simulink model "sst"  (R2025a)
settings: Solver=ode1be  StartTime=0.0  StopTime=simlength  FixedStep=tc  MaxStep=ts_sim
values from neighbouring files (symbols this model uses):
  Adrso = eye(2) + Arso*ts_inv    [design_model.m]
  alpha = 35    [design_model.m]
  C1 = 0.5    [design_model.m]
  Crso = [1 0]    [design_model.m]
  DThs_init = 0    [design_model.m]
  E0 = 3.485    [design_model.m]
  E1 = 0.2156    [design_model.m]
  E2 = 0    [design_model.m]
  E3 = 0    [design_model.m]
  E_1 = -1.031    [design_model.m]
  Elog = -0.05    [design_model.m]
  fPWM_DAB = fPWM_INV    (= 35000)    [design_model.m]
  fPWM_INV = 35e3    (= 35000)    [design_model.m]
  freq = 50    [design_model.m]
  I_FS = Iout_ac_rms_nom * sqrt(2) * margin_factor    [design_model.m]
  ki_i_dab = 18    [design_model.m]
  ki_pll = 3140    [design_model.m]
  ki_v_dab = 45    [design_model.m]
  kp_i_dab = 2    [design_model.m]
  kp_pll = 314    [design_model.m]
  kp_v_dab = 8    [design_model.m]
  Ldrso = acker(Adrso',Crso',polesdrso)'    [design_model.m]
  M = 125    [design_model.m]
  number_of_cells = 30    [design_model.m]
  Q = 1000    [design_model.m]
  q1Kalman = ts_inv^2    (= 8.16326530612e-10)    [design_model.m]
  q2Kalman = ts_inv^1    (= 2.85714285714e-05)    [design_model.m]
  q3Kalman = 0    [design_model.m]
  R0 = 0.0035    [design_model.m]
  R1 = 0.0035    [design_model.m]
  rKalman = 1    [design_model.m]
  Tambient = 40    [design_model.m]
  tc = ts_inv/200    (= 1.42857142857e-07)    [design_model.m]
  ts_afe = ts_inv    (= 2.85714285714e-05)    [design_model.m]
  ts_dab = tPWM_DAB*2    (= 5.71428571429e-05)    [design_model.m]
  ts_inv = tPWM_INV    (= 2.85714285714e-05)    [design_model.m]
  V_FS = Vout_dc_nom * margin_factor    (= 500)    [design_model.m]
  weigth = 0.6/6    (= 0.1)    [design_model.m]
undefined symbols (not defined in the file or in its folder): Aresd, Bresd, Cresd, dead_time_DAB, dead_time_INV, iph_grid_pu_ref, ki_afe, kp_afe, LFu1_AFE, n_modules, omega_grid_nom, RLFu1_AFE, ts_battery, tsample, V_phase_normalization_factor, Vdab2_dc_nom
libraries: fl_lib x280, nesl_utility x188, ee_lib x41, cstblocks x4, single_phase_transformer_lib x2, lithium_ion_cell_lib x1, simulink x1
(part 1 of 12)
settings Model: SimulationMode=accelerator  Creator=LTNBDA  LastModifiedBy=dbagn
settings SolverCC: ZeroCrossControl=EnableAll  ZeroCrossAlgorithm=Adaptive  AlgebraicLoopSolver=TrustRegion  SolverResetMethod=Robust  AutoInsertRateTranBlk=on
settings DataIOCC: LimitDataPoints=on  MaxDataPoints=1  SaveFormat=Array  SignalLoggingSaveFormat=ModelDataLogs  SaveOutput=off  SignalLogging=off  DSMLogging=off  SaveTime=off  ReturnWorkspaceOutputs=off
settings OptimizationCC: ExpressionDepthLimit=2147483647.0  InitFltsAndDblsToZero=on  EfficientMapNaN2IntZero=off  LifeSpan=inf
settings DebuggingCC: SaveWithParameterizedLinksMsg=none  UnderspecifiedInitializationDetection=Classic  MergeDetectMultiDrivingBlocksExec=none  SignalResolutionControl=TryResolveAllWithWarning  SolverPrmCheckMsg=warning  MultiTaskDSMMsg=warning  MultiTaskCondExecSysMsg=none  MultiTaskRateTransMsg=warning  FcnCallInpInsideContextMsg=warning  StateNameClashWarn=warning  SFUnexpectedBacktrackingDiag=warning  SFNoUnconditionalDefaultTransitionDiag=warning  ArithmeticOperatorsInVariantConditions=warning
settings HardwareCC: ProdBitPerLong=64.0  ProdLargestAtomicFloat=None  ProdIntDivRoundTo=Undefined  ProdEndianess=Unspecified  ProdHWDeviceType=Generic->64-bit Embedded Processor (LP64)  TargetBitPerPointer=64.0  TargetBitPerSizeT=64.0  TargetBitPerPtrDiffT=64.0  TargetLongLongMode=on  TargetIntDivRoundTo=Zero  TargetEndianess=LittleEndian  TargetWordSize=64.0  TargetHWDeviceType=MATLAB Host  ProdEqTarget=off
settings ModelReferenceCC: EnableRefExpFcnMdlSchedulingChecks=on  PropagateSignalLabelsOutOfModel=off
settings SFSimCC: SimUseLocalCustomCode=off  CustomCodeUndefinedFunction=UseInterfaceOnly
settings RTWCC: RTWUseLocalCustomCode=off  GPUComputeCapability=3.5
settings CodeAppCC: MaxIdLength=128.0  StateflowObjectComments=on
settings GRTTargetCC: TargetLangStandard=C89/C90 (ANSI)  CombineOutputUpdateFcns=off  GRTInterface=on
settings ConfigComp: CovMetricSettings=dw  CovSaveCumulativeToWorkspaceVar=on  CovSaveSingleToWorkspaceVar=on  CovExternalEMLEnable=off
settings SimscapeCC: SimscapeNormalizeSystem=off

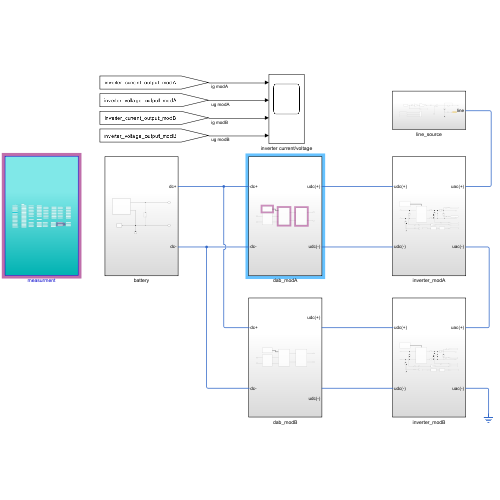
[thumbnail: Simulink's stored preview of the top-level diagram]
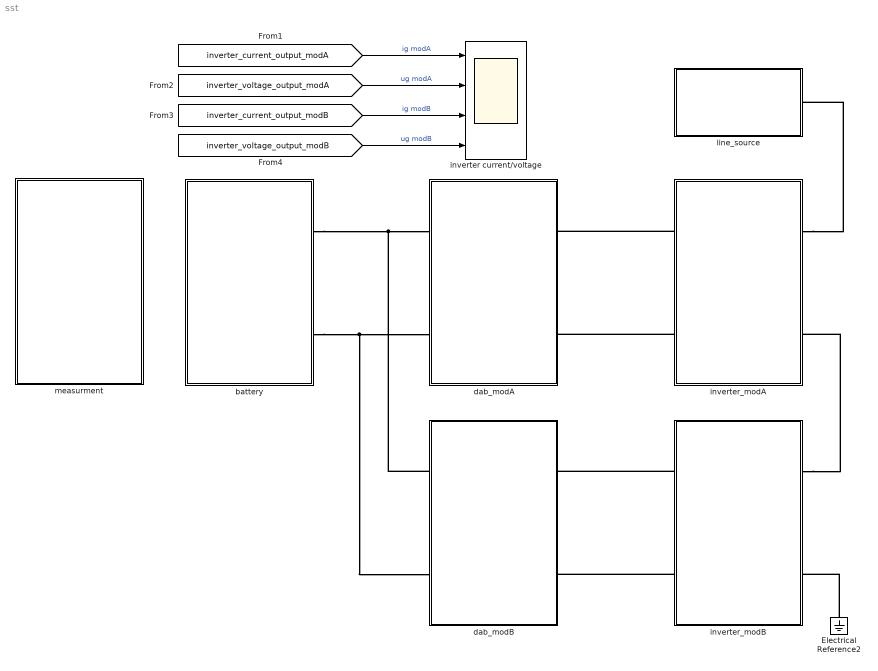
== system sst ==
  Electrical Reference2 : fl_lib/Electrical/Electrical Elements/Electrical Reference
  battery : Subsystem
  dab_modA : Subsystem
  dab_modB : Subsystem
  inverter current/voltage : Scope  NumInputPorts=4
      settings: SampleTime=tc  ActiveDisplayYMinimum=-1010.1784758110234  ActiveDisplayYMaximum=2328.1180145143348
  inverter_modA : Subsystem
  inverter_modB : Subsystem
  line_source : Subsystem
  measurment : Subsystem
  wires:
  [inverter_current_output_modA] -> inverter current/voltage/1  "ig modA"
  [inverter_voltage_output_modA] -> inverter current/voltage/2  "ug modA"
  [inverter_current_output_modB] -> inverter current/voltage/3  "ig modB"
  [inverter_voltage_output_modB] -> inverter current/voltage/4  "ug modB"
  connections:
  inverter_modA/LConn2 -- dab_modA/RConn2
  inverter_modA/LConn1 -- dab_modA/RConn1
  inverter_modA/RConn1 -- line_source/LConn1
  battery/RConn1 -- dab_modB/LConn1 -- dab_modA/LConn1
  battery/RConn2 -- dab_modB/LConn2 -- dab_modA/LConn2
  inverter_modB/LConn1 -- dab_modB/RConn1
  inverter_modB/LConn2 -- dab_modB/RConn2
  Electrical Reference2/LConn1 -- inverter_modB/RConn2
  inverter_modB/RConn1 -- inverter_modA/RConn2

== system sst/battery ==
  Electrical Reference1 : fl_lib/Electrical/Electrical Elements/Electrical Reference
  LithiumIonBattery : Subsystem
  Solver Configuration : nesl_utility/Solver Configuration  PhysicalDomain=network_engine_domain  SubClassName=solver  LeftPortType=input  RightPortType=generic  Tones=[]  Harmonics=[]  SimulateNoise=off  Profile=off  UseLocalSampling=off  EnableSwitchedLinearOptims=on  FrequencyDomain=off  UseCCode=off  RelTol=0.001  AbsTol=0.001  MinStep=1e-09  ToWorkspace=off  RevertToSquareIcSolve=off  NumHomotopyIterations=100  PhasorMode=off  PhasorModeNumHarmonics=1  ConsistencySolver=NEWTON_FTOL  IndexReductionMethod=DerivativeReplacement  DoDC=on  ResidualTolerance=1e-09  ConsistencyTolSource=GLOBAL  ConsistencyAbsTol=0.001  ConsistencyRelTol=0.001  ConsistencyTolFactor=0.001  UseLocalSolver=on  LocalSolverChoice=NE_BACKWARD_EULER_ADVANCER  ResolveIndetEquations=on  FunctionEvalNumThread=1  LocalSolverSampleTime=tc  DoFixedCost=on  MaxNonlinIter=3  MaxModeIter=2  ComputeImpulses=off  ImpulseIterations=2  LinearAlgebra=auto  LinearAlgebraNumThread=0  EquationFormulation=NE_TIME_EF  DelaysMemoryBudget=1024  AutomaticFiltering=on  FilteringTimeConstant=0.001  PartitionStorageMethod=AS_NEEDED  PartitionMemoryBudget=1024  PartitionMethod=ROBUST  MultibodyUseLocalSolver=off  MultibodyLocalSolverChoice=ODE1  MultibodyLocalSolverSampleTime=0.001
  Voltage Source : ee_lib/Sources/Voltage Source  Commented=on  dc_voltage=ubattery V  ac_voltage=0 V  ac_shift=0 rad  ac_frequency=60 Hz  noise_mode=ee.enum.sources.noise.Disabled  PSD=0 V^2/Hz  sample_time=1e-3 s  repeatability=ee.enum.sources.repeatability.NotRepeatable  user_seed=0  auto_seed=3499211588  i_specify=off  i_priority=None  i=0 A  i_nominal_specify=off  i_nominal_value=1  i_nominal_unit=A  v_specify=off  v_priority=None  v=0 V  v_nominal_specify=off  v_nominal_value=1  v_nominal_unit=V
  dc+ : PMIOPort  Side=Right
  dc- : PMIOPort  Port=2  Side=Right
  connections:
  Voltage Source/RConn1 -- LithiumIonBattery/RConn2 -- Electrical Reference1/LConn1 -- Solver Configuration/RConn1 -- dc-/RConn1
  Voltage Source/LConn1 -- LithiumIonBattery/RConn1 -- dc+/RConn1

== system sst/dab_modA ==
  dab_ctrl : Subsystem
  dc/dc with galvanic isolation : Subsystem
  single_phase_ui_measure1 : Subsystem
  ui_measure : Subsystem
  udc(+) : PMIOPort  Side=Right
  udc(-) : PMIOPort  Port=2  Side=Right
  dc+ : PMIOPort  Port=3  Side=Left
  dc- : PMIOPort  Port=4  Side=Left
  wires:
  dab_ctrl/1(gate_commands) -> dc/dc with galvanic isolation/1(gate_commands)
  connections:
  dc/dc with galvanic isolation/RConn1 -- ui_measure/LConn1
  dc/dc with galvanic isolation/RConn2 -- ui_measure/LConn2
  udc(+)/RConn1 -- ui_measure/RConn1
  udc(-)/RConn1 -- ui_measure/RConn2
  dc/dc with galvanic isolation/LConn2 -- single_phase_ui_measure1/RConn2
  single_phase_ui_measure1/RConn1 -- dc/dc with galvanic isolation/LConn1
  dc+/RConn1 -- single_phase_ui_measure1/LConn1
  dc-/RConn1 -- single_phase_ui_measure1/LConn2

== system sst/dab_modB ==
  dab_ctrl : Subsystem
  dc/dc with galvanic isolation : Subsystem
  single_phase_ui_measure1 : Subsystem
  ui_measure : Subsystem
  udc(+) : PMIOPort  Side=Right
  udc(-) : PMIOPort  Port=2  Side=Right
  dc+ : PMIOPort  Port=3  Side=Left
  dc- : PMIOPort  Port=4  Side=Left
  wires:
  dab_ctrl/1(gate_commands) -> dc/dc with galvanic isolation/1(gate_commands)
  connections:
  dc-/RConn1 -- single_phase_ui_measure1/LConn2
  dc+/RConn1 -- single_phase_ui_measure1/LConn1
  single_phase_ui_measure1/RConn1 -- dc/dc with galvanic isolation/LConn1
  dc/dc with galvanic isolation/LConn2 -- single_phase_ui_measure1/RConn2
  udc(-)/RConn1 -- ui_measure/RConn2
  udc(+)/RConn1 -- ui_measure/RConn1
  dc/dc with galvanic isolation/RConn2 -- ui_measure/LConn2
  dc/dc with galvanic isolation/RConn1 -- ui_measure/LConn1

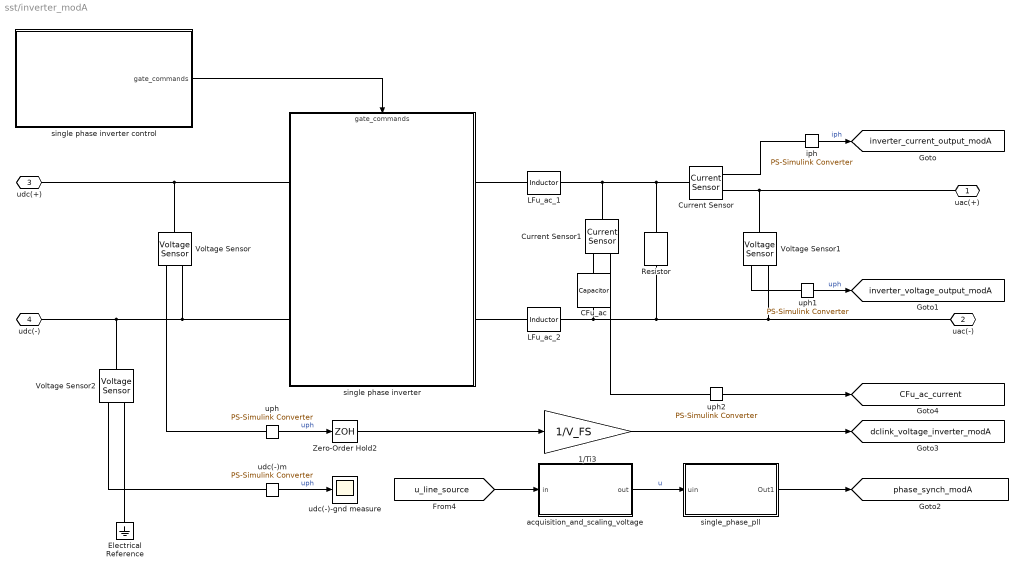
== system sst/inverter_modA ==
  1/Ti3 : Gain  Gain=1/V_FS  SaturateOnIntegerOverflow=on  OutDataTypeStr=Inherit: Same as input  ParamDataTypeStr=Inherit: Same as input
  CFu_ac : fl_lib/Electrical/Electrical Elements/Capacitor  c=CFu_AFE F  r=RCFu_AFE Ohm  g=0 1/Ohm  i_specify=off  i_priority=None  i=0 A  i_nominal_specify=off  i_nominal_value=1  i_nominal_unit=A  v_specify=off  v_priority=None  v=0 V  v_nominal_specify=off  v_nominal_value=1  v_nominal_unit=V  vc_specify=off  vc_priority=High  vc=0 V  vc_nominal_specify=off  vc_nominal_value=1  vc_nominal_unit=V
  Current Sensor : fl_lib/Electrical/Electrical Sensors/Current Sensor
  Current Sensor1 : fl_lib/Electrical/Electrical Sensors/Current Sensor
  Electrical Reference : fl_lib/Electrical/Electrical Elements/Electrical Reference
  LFu_ac_1 : fl_lib/Electrical/Electrical Elements/Inductor  l=LFu1_AFE/2 H  r=RLFu1_AFE/2 Ohm  g=0 1/Ohm  i_specify=off  i_priority=None  i=0 A  i_nominal_specify=off  i_nominal_value=1  i_nominal_unit=A  v_specify=off  v_priority=None  v=0 V  v_nominal_specify=off  v_nominal_value=1  v_nominal_unit=V  i_L_specify=off  i_L_priority=High  i_L=0 A  i_L_nominal_specify=off  i_L_nominal_value=1  i_L_nominal_unit=A
  LFu_ac_2 : fl_lib/Electrical/Electrical Elements/Inductor  l=LFu1_AFE/2 H  r=RLFu1_AFE/2 Ohm  g=0 1/Ohm  i_specify=off  i_priority=None  i=0 A  i_nominal_specify=off  i_nominal_value=1  i_nominal_unit=A  v_specify=off  v_priority=None  v=0 V  v_nominal_specify=off  v_nominal_value=1  v_nominal_unit=V  i_L_specify=off  i_L_priority=High  i_L=0 A  i_L_nominal_specify=off  i_L_nominal_value=1  i_L_nominal_unit=A
  Resistor : fl_lib/Electrical/Electrical Elements/Resistor  R=10e3 Ohm  i_specify=off  i_priority=None  i=0 A  i_nominal_specify=off  i_nominal_value=1  i_nominal_unit=A  v_specify=off  v_priority=None  v=0 V  v_nominal_specify=off  v_nominal_value=1  v_nominal_unit=V
  Voltage Sensor : fl_lib/Electrical/Electrical Sensors/Voltage Sensor
  Voltage Sensor1 : fl_lib/Electrical/Electrical Sensors/Voltage Sensor
  Voltage Sensor2 : fl_lib/Electrical/Electrical Sensors/Voltage Sensor
  Zero-Order Hold2 : ZeroOrderHold  SampleTime=ts_inv
  acquisition_and_scaling_voltage : Subsystem
  iph : nesl_utility/PS-Simulink Converter  PhysicalDomain=network_engine_domain  SubClassName=ps_output  LeftPortType=input  RightPortType=output  PseudoPeriodic=off  Frequencies=[]  VectorFormat=1-D array  Unit=A  AffineConversion=off
  single phase inverter : Subsystem
      settings: PortSchema="{\"entries\":[{\"content\":{\"sides\":[{\"content\":{\"connectorIds\":[\"LConn1\",\"LConn2\"]},\"type\":\"ConnectorPlacement.EquallySpacedRectSide\",\"uuid\":\"4fcf4fea-d38f-431b-8a91-be3ce9782faf\"},{\"content\":{\"connectorIds\":[\"RConn1\",\"RConn2\"],\"side\":\"RIGHT\"},\"type\":\"ConnectorPlacement.EquallySpacedRectSide\",\"uuid\":\"0aa56277-92e9-4e3b-84c7-43398254a4d8\"},{\"content\":{\"connectorIds\":[\"In1\"],\"side\":\"TOP\"},\"type\":\"ConnectorPlacement.EquallySpacedRectSide\",\"uuid\":\"5cd150dc-bcaf-4cd7-b2a8-3db203726730\"}]},\"type\":\"ConnectorPlacement.EquallySpacedConnector\",\"uuid\":\"bf8194c4-c327-4d40-bea4-f1e7617f80b4\"}],\"packageUris\":[\"http://schema.mathworks.com/mf0/Connector/R2020b\"],\"version\":\"1.0\"}"
  single phase inverter control : Subsystem
  single_phase_pll : Subsystem
  udc(-)-gnd measure : Scope
      settings: SampleTime=tc  ActiveDisplayYMinimum=-538.53095  ActiveDisplayYMaximum=99.4357
  udc(-)m : nesl_utility/PS-Simulink Converter  PhysicalDomain=network_engine_domain  SubClassName=ps_output  LeftPortType=input  RightPortType=output  PseudoPeriodic=off  Frequencies=[]  VectorFormat=1-D array  Unit=V  AffineConversion=off
  uph : nesl_utility/PS-Simulink Converter  PhysicalDomain=network_engine_domain  SubClassName=ps_output  LeftPortType=input  RightPortType=output  PseudoPeriodic=off  Frequencies=[]  VectorFormat=1-D array  Unit=V  AffineConversion=off
  uph1 : nesl_utility/PS-Simulink Converter  PhysicalDomain=network_engine_domain  SubClassName=ps_output  LeftPortType=input  RightPortType=output  PseudoPeriodic=off  Frequencies=[]  VectorFormat=1-D array  Unit=V  AffineConversion=off
  uph2 : nesl_utility/PS-Simulink Converter  PhysicalDomain=network_engine_domain  SubClassName=ps_output  LeftPortType=input  RightPortType=output  PseudoPeriodic=off  Frequencies=[]  VectorFormat=1-D array  Unit=A  AffineConversion=off
  uac(+) : PMIOPort  Side=Right
  uac(-) : PMIOPort  Port=2  Side=Right
  udc(+) : PMIOPort  Port=3  Side=Left
  udc(-) : PMIOPort  Port=4  Side=Left
  tag scope: CFu_ac_current=global, dclink_voltage_inverter_modA=global, inverter_current_output_modA=global, inverter_voltage_output_modA=global, phase_synch_modA=global
  wires:
  Zero-Order Hold2/1 -> 1/Ti3/1
  1/Ti3/1 -> [dclink_voltage_inverter_modA]
  single phase inverter control/1(gate_commands) -> single phase inverter/1(gate_commands)
  uph/1 -> Zero-Order Hold2/1  "uph"
  iph/1 -> [inverter_current_output_modA]  "iph"
  uph1/1 -> [inverter_voltage_output_modA]  "uph"
  udc(-)m/1 -> udc(-)-gnd measure/1  "uph"
  uph2/1 -> [CFu_ac_current]
  acquisition_and_scaling_voltage/1(out) -> single_phase_pll/1(uin)  "u"
  [u_line_source] -> acquisition_and_scaling_voltage/1(in)
  single_phase_pll/1(Out1) -> [phase_synch_modA]
  connections:
  single phase inverter/RConn2 -- Voltage Sensor/RConn2 -- Voltage Sensor2/LConn1 -- udc(-)/RConn1
  single phase inverter/RConn1 -- Voltage Sensor/LConn1 -- udc(+)/RConn1
  LFu_ac_1/LConn1 -- single phase inverter/LConn1
  single phase inverter/LConn2 -- LFu_ac_2/RConn1
  Voltage Sensor/RConn1 -- uph/LConn1
  Voltage Sensor1/RConn1 -- uph1/LConn1
  Electrical Reference/LConn1 -- Voltage Sensor2/RConn2
  Voltage Sensor2/RConn1 -- udc(-)m/LConn1
  Resistor/LConn1 -- Current Sensor/LConn1 -- Current Sensor1/LConn1 -- LFu_ac_1/RConn1
  iph/LConn1 -- Current Sensor/RConn1
  uac(+)/RConn1 -- Current Sensor/RConn2 -- Voltage Sensor1/LConn1
  LFu_ac_2/LConn1 -- uac(-)/RConn1 -- Voltage Sensor1/RConn2 -- Resistor/RConn1 -- CFu_ac/RConn1
  Current Sensor1/RConn2 -- CFu_ac/LConn1
  Current Sensor1/RConn1 -- uph2/LConn1

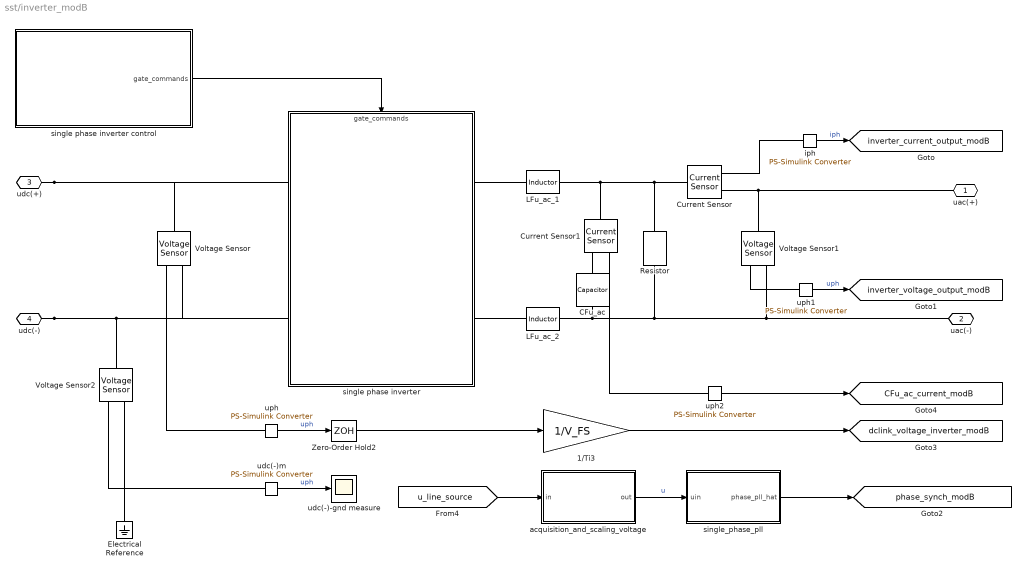
== system sst/inverter_modB ==
  1/Ti3 : Gain  Gain=1/V_FS  SaturateOnIntegerOverflow=on  OutDataTypeStr=Inherit: Same as input  ParamDataTypeStr=Inherit: Same as input
  CFu_ac : fl_lib/Electrical/Electrical Elements/Capacitor  c=CFu_AFE F  r=RCFu_AFE Ohm  g=0 1/Ohm  i_specify=off  i_priority=None  i=0 A  i_nominal_specify=off  i_nominal_value=1  i_nominal_unit=A  v_specify=off  v_priority=None  v=0 V  v_nominal_specify=off  v_nominal_value=1  v_nominal_unit=V  vc_specify=off  vc_priority=High  vc=0 V  vc_nominal_specify=off  vc_nominal_value=1  vc_nominal_unit=V
  Current Sensor : fl_lib/Electrical/Electrical Sensors/Current Sensor
  Current Sensor1 : fl_lib/Electrical/Electrical Sensors/Current Sensor
  Electrical Reference : fl_lib/Electrical/Electrical Elements/Electrical Reference
  LFu_ac_1 : fl_lib/Electrical/Electrical Elements/Inductor  l=LFu1_AFE/2 H  r=RLFu1_AFE/2 Ohm  g=0 1/Ohm  i_specify=off  i_priority=None  i=0 A  i_nominal_specify=off  i_nominal_value=1  i_nominal_unit=A  v_specify=off  v_priority=None  v=0 V  v_nominal_specify=off  v_nominal_value=1  v_nominal_unit=V  i_L_specify=off  i_L_priority=High  i_L=0 A  i_L_nominal_specify=off  i_L_nominal_value=1  i_L_nominal_unit=A
  LFu_ac_2 : fl_lib/Electrical/Electrical Elements/Inductor  l=LFu1_AFE/2 H  r=RLFu1_AFE/2 Ohm  g=0 1/Ohm  i_specify=off  i_priority=None  i=0 A  i_nominal_specify=off  i_nominal_value=1  i_nominal_unit=A  v_specify=off  v_priority=None  v=0 V  v_nominal_specify=off  v_nominal_value=1  v_nominal_unit=V  i_L_specify=off  i_L_priority=High  i_L=0 A  i_L_nominal_specify=off  i_L_nominal_value=1  i_L_nominal_unit=A
  Resistor : fl_lib/Electrical/Electrical Elements/Resistor  R=10e3 Ohm  i_specify=off  i_priority=None  i=0 A  i_nominal_specify=off  i_nominal_value=1  i_nominal_unit=A  v_specify=off  v_priority=None  v=0 V  v_nominal_specify=off  v_nominal_value=1  v_nominal_unit=V
  Voltage Sensor : fl_lib/Electrical/Electrical Sensors/Voltage Sensor
  Voltage Sensor1 : fl_lib/Electrical/Electrical Sensors/Voltage Sensor
  Voltage Sensor2 : fl_lib/Electrical/Electrical Sensors/Voltage Sensor
  Zero-Order Hold2 : ZeroOrderHold  SampleTime=ts_inv
  acquisition_and_scaling_voltage : Subsystem
  iph : nesl_utility/PS-Simulink Converter  PhysicalDomain=network_engine_domain  SubClassName=ps_output  LeftPortType=input  RightPortType=output  PseudoPeriodic=off  Frequencies=[]  VectorFormat=1-D array  Unit=A  AffineConversion=off
  single phase inverter : Subsystem
      settings: PortSchema="{\"entries\":[{\"content\":{\"sides\":[{\"content\":{\"connectorIds\":[\"LConn1\",\"LConn2\"]},\"type\":\"ConnectorPlacement.EquallySpacedRectSide\",\"uuid\":\"4fcf4fea-d38f-431b-8a91-be3ce9782faf\"},{\"content\":{\"connectorIds\":[\"RConn1\",\"RConn2\"],\"side\":\"RIGHT\"},\"type\":\"ConnectorPlacement.EquallySpacedRectSide\",\"uuid\":\"0aa56277-92e9-4e3b-84c7-43398254a4d8\"},{\"content\":{\"connectorIds\":[\"In1\"],\"side\":\"TOP\"},\"type\":\"ConnectorPlacement.EquallySpacedRectSide\",\"uuid\":\"5cd150dc-bcaf-4cd7-b2a8-3db203726730\"}]},\"type\":\"ConnectorPlacement.EquallySpacedConnector\",\"uuid\":\"bf8194c4-c327-4d40-bea4-f1e7617f80b4\"}],\"packageUris\":[\"http://schema.mathworks.com/mf0/Connector/R2020b\"],\"version\":\"1.0\"}"
  single phase inverter control : Subsystem
  single_phase_pll : Subsystem
  udc(-)-gnd measure : Scope
      settings: SampleTime=tc  ActiveDisplayYMinimum=-25903.27191628638  ActiveDisplayYMaximum=4545.99688176282
  udc(-)m : nesl_utility/PS-Simulink Converter  PhysicalDomain=network_engine_domain  SubClassName=ps_output  LeftPortType=input  RightPortType=output  PseudoPeriodic=off  Frequencies=[]  VectorFormat=1-D array  Unit=V  AffineConversion=off
  uph : nesl_utility/PS-Simulink Converter  PhysicalDomain=network_engine_domain  SubClassName=ps_output  LeftPortType=input  RightPortType=output  PseudoPeriodic=off  Frequencies=[]  VectorFormat=1-D array  Unit=V  AffineConversion=off
  uph1 : nesl_utility/PS-Simulink Converter  PhysicalDomain=network_engine_domain  SubClassName=ps_output  LeftPortType=input  RightPortType=output  PseudoPeriodic=off  Frequencies=[]  VectorFormat=1-D array  Unit=V  AffineConversion=off
  uph2 : nesl_utility/PS-Simulink Converter  PhysicalDomain=network_engine_domain  SubClassName=ps_output  LeftPortType=input  RightPortType=output  PseudoPeriodic=off  Frequencies=[]  VectorFormat=1-D array  Unit=A  AffineConversion=off
  uac(+) : PMIOPort  Side=Right
  uac(-) : PMIOPort  Port=2  Side=Right
  udc(+) : PMIOPort  Port=3  Side=Left
  udc(-) : PMIOPort  Port=4  Side=Left
  tag scope: CFu_ac_current_modB=global, dclink_voltage_inverter_modB=global, inverter_current_output_modB=global, inverter_voltage_output_modB=global, phase_synch_modB=global
  wires:
  single_phase_pll/1(phase_pll_hat) -> [phase_synch_modB]
  [u_line_source] -> acquisition_and_scaling_voltage/1(in)
  acquisition_and_scaling_voltage/1(out) -> single_phase_pll/1(uin)  "u"
  uph2/1 -> [CFu_ac_current_modB]
  udc(-)m/1 -> udc(-)-gnd measure/1  "uph"
  uph1/1 -> [inverter_voltage_output_modB]  "uph"
  iph/1 -> [inverter_current_output_modB]  "iph"
  uph/1 -> Zero-Order Hold2/1  "uph"
  single phase inverter control/1(gate_commands) -> single phase inverter/1(gate_commands)
  1/Ti3/1 -> [dclink_voltage_inverter_modB]
  Zero-Order Hold2/1 -> 1/Ti3/1
  connections:
  Current Sensor1/RConn1 -- uph2/LConn1
  Current Sensor1/RConn2 -- CFu_ac/LConn1
  CFu_ac/RConn1 -- Resistor/RConn1 -- Voltage Sensor1/RConn2 -- uac(-)/RConn1 -- LFu_ac_2/LConn1
  Voltage Sensor1/LConn1 -- Current Sensor/RConn2 -- uac(+)/RConn1
  iph/LConn1 -- Current Sensor/RConn1
  LFu_ac_1/RConn1 -- Current Sensor1/LConn1 -- Current Sensor/LConn1 -- Resistor/LConn1
  Voltage Sensor2/RConn1 -- udc(-)m/LConn1
  Electrical Reference/LConn1 -- Voltage Sensor2/RConn2
  Voltage Sensor1/RConn1 -- uph1/LConn1
  Voltage Sensor/RConn1 -- uph/LConn1
  single phase inverter/LConn2 -- LFu_ac_2/RConn1
  LFu_ac_1/LConn1 -- single phase inverter/LConn1
  udc(+)/RConn1 -- Voltage Sensor/LConn1 -- single phase inverter/RConn1
  udc(-)/RConn1 -- Voltage Sensor2/LConn1 -- Voltage Sensor/RConn2 -- single phase inverter/RConn2

== system sst/line_source ==
  Controlled Voltage Source : fl_lib/Electrical/Electrical Sources/Controlled Voltage Source
  Cos : Trigonometry  Operator=cos
  Electrical Reference : fl_lib/Electrical/Electrical Elements/Electrical Reference
  Electrical Reference1 : fl_lib/Electrical/Electrical Elements/Electrical Reference
  Gain : Gain  Gain=V_phase_normalization_factor
  Gain1 : Gain  Gain=n_modules
  Ld_grid : fl_lib/Electrical/Electrical Elements/Inductor  l=Ld2_trafo H  r=3e-3 Ohm  g=0 1/Ohm  i_specify=off  i_priority=None  i=0 A  i_nominal_specify=off  i_nominal_value=1  i_nominal_unit=A  v_specify=off  v_priority=None  v=0 V  v_nominal_specify=off  v_nominal_value=1  v_nominal_unit=V  i_L_specify=off  i_L_priority=High  i_L=0 A  i_L_nominal_specify=off  i_L_nominal_value=1  i_L_nominal_unit=A
  Simulink-PS Converter : nesl_utility/Simulink-PS Converter  PhysicalDomain=network_engine_domain  SubClassName=ps_input  LeftPortType=input  RightPortType=output  PseudoPeriodic=off  Frequencies=[]  NoiseDistribution=none  NoiseParameters=[]  Unit=1  AffineConversion=off  FilteringAndDerivatives=provide  SimscapeFilterOrder=1  InputFilterTimeConstant=0.001  UdotUserProvided=0
  Voltage Sensor2 : fl_lib/Electrical/Electrical Sensors/Voltage Sensor
  phase_gen : Subsystem
  phase_grid/pll : Scope  NumInputPorts=3
      settings: SampleTime=tc  ActiveDisplayYMinimum=-3.92515736330459  ActiveDisplayYMaximum=3.9104897338435562
  u_line_source : nesl_utility/PS-Simulink Converter  PhysicalDomain=network_engine_domain  SubClassName=ps_output  LeftPortType=input  RightPortType=output  PseudoPeriodic=off  Frequencies=[]  VectorFormat=1-D array  Unit=V  AffineConversion=off
  line : PMIOPort  Side=Left
  tag scope: phase_grid=global, u_line_source=global
  wires:
  phase_gen/1(phase_gen) -> Cos/1, [phase_grid]
  Cos/1 -> Gain1/1
  Gain/1 -> Simulink-PS Converter/1
  [phase_synch_modA] -> phase_grid/pll/1  "phase_synch_modA"
  [phase_grid] -> phase_grid/pll/2  "phase_grid"
  u_line_source/1 -> [u_line_source]  "u_line_source"
  Gain1/1 -> Gain/1
  [phase_synch_modB] -> phase_grid/pll/3  "phase_synch_modB"
  connections:
  Simulink-PS Converter/RConn1 -- Controlled Voltage Source/RConn1
  Controlled Voltage Source/LConn1 -- Ld_grid/LConn1
  Voltage Sensor2/RConn1 -- u_line_source/LConn1
  Electrical Reference1/LConn1 -- Voltage Sensor2/RConn2
  Controlled Voltage Source/RConn2 -- Electrical Reference/LConn1
  Ld_grid/RConn1 -- line/RConn1 -- Voltage Sensor2/LConn1

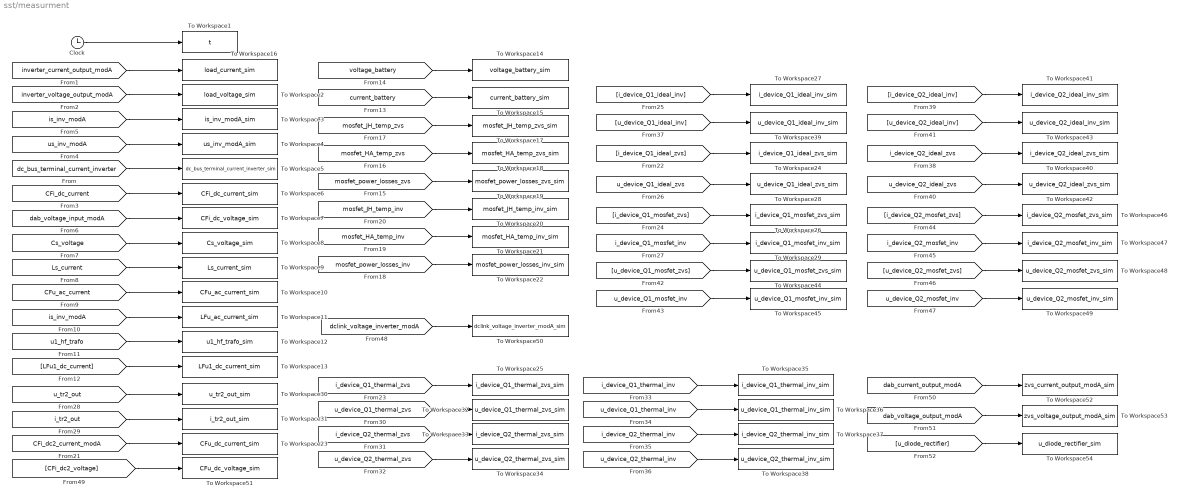
== system sst/measurment ==
  Clock : Clock
  To Workspace1 : ToWorkspace  VariableName=t  SampleTime=tc
      settings: MaxDataPoints=Nc
  To Workspace10 : ToWorkspace  VariableName=CFu_ac_current_sim  SampleTime=tc
      settings: MaxDataPoints=Nc
  To Workspace11 : ToWorkspace  VariableName=LFu_ac_current_sim  SampleTime=tc
      settings: MaxDataPoints=Nc
  To Workspace12 : ToWorkspace  VariableName=u1_hf_trafo_sim  SampleTime=tc
      settings: MaxDataPoints=Nc
  To Workspace13 : ToWorkspace  VariableName=LFu1_dc_current_sim  SampleTime=tc
      settings: MaxDataPoints=Nc
  To Workspace14 : ToWorkspace  VariableName=voltage_battery_sim  SampleTime=tc
      settings: MaxDataPoints=Nc
  To Workspace15 : ToWorkspace  VariableName=current_battery_sim  SampleTime=tc
      settings: MaxDataPoints=Nc
  To Workspace16 : ToWorkspace  VariableName=load_current_sim  SampleTime=tc
      settings: MaxDataPoints=Nc
  To Workspace17 : ToWorkspace  VariableName=mosfet_JH_temp_zvs_sim  SampleTime=tc
      settings: MaxDataPoints=Nc
  To Workspace18 : ToWorkspace  VariableName=mosfet_HA_temp_zvs_sim  SampleTime=tc
      settings: MaxDataPoints=Nc
  To Workspace19 : ToWorkspace  VariableName=mosfet_power_losses_zvs_sim  SampleTime=tc
      settings: MaxDataPoints=Nc
  To Workspace2 : ToWorkspace  VariableName=load_voltage_sim  SampleTime=tc
      settings: MaxDataPoints=Nc
  To Workspace20 : ToWorkspace  VariableName=mosfet_JH_temp_inv_sim  SampleTime=tc
      settings: MaxDataPoints=Nc
  To Workspace21 : ToWorkspace  VariableName=mosfet_HA_temp_inv_sim  SampleTime=tc
      settings: MaxDataPoints=Nc
  To Workspace22 : ToWorkspace  VariableName=mosfet_power_losses_inv_sim  SampleTime=tc
      settings: MaxDataPoints=Nc
  To Workspace23 : ToWorkspace  VariableName=CFu_dc_current_sim  SampleTime=tc
      settings: MaxDataPoints=Nc
  To Workspace24 : ToWorkspace  VariableName=i_device_Q1_ideal_zvs_sim  SampleTime=tc
      settings: MaxDataPoints=Nc
  To Workspace25 : ToWorkspace  VariableName=i_device_Q1_thermal_zvs_sim  SampleTime=tc
      settings: MaxDataPoints=Nc
  To Workspace26 : ToWorkspace  VariableName=i_device_Q1_mosfet_zvs_sim  SampleTime=tc
      settings: MaxDataPoints=Nc
  To Workspace27 : ToWorkspace  VariableName=i_device_Q1_ideal_inv_sim  SampleTime=tc
      settings: MaxDataPoints=Nc
  To Workspace28 : ToWorkspace  VariableName=u_device_Q1_ideal_zvs_sim  SampleTime=tc
      settings: MaxDataPoints=Nc
  To Workspace29 : ToWorkspace  VariableName=i_device_Q1_mosfet_inv_sim  SampleTime=tc
      settings: MaxDataPoints=Nc
  To Workspace3 : ToWorkspace  VariableName=is_inv_modA_sim  SampleTime=tc
      settings: MaxDataPoints=Nc
  To Workspace30 : ToWorkspace  VariableName=u_tr2_out_sim  SampleTime=tc
      settings: MaxDataPoints=Nc
  To Workspace31 : ToWorkspace  VariableName=i_tr2_out_sim  SampleTime=tc
      settings: MaxDataPoints=Nc
  To Workspace32 : ToWorkspace  VariableName=u_device_Q1_thermal_zvs_sim  SampleTime=tc
      settings: MaxDataPoints=Nc
  To Workspace33 : ToWorkspace  VariableName=i_device_Q2_thermal_zvs_sim  SampleTime=tc
      settings: MaxDataPoints=Nc
  To Workspace34 : ToWorkspace  VariableName=u_device_Q2_thermal_zvs_sim  SampleTime=tc
      settings: MaxDataPoints=Nc
  To Workspace35 : ToWorkspace  VariableName=i_device_Q1_thermal_inv_sim  SampleTime=tc
      settings: MaxDataPoints=Nc
  To Workspace36 : ToWorkspace  VariableName=u_device_Q1_thermal_inv_sim  SampleTime=tc
      settings: MaxDataPoints=Nc
  To Workspace37 : ToWorkspace  VariableName=i_device_Q2_thermal_inv_sim  SampleTime=tc
      settings: MaxDataPoints=Nc
  To Workspace38 : ToWorkspace  VariableName=u_device_Q2_thermal_inv_sim  SampleTime=tc
      settings: MaxDataPoints=Nc
  To Workspace39 : ToWorkspace  VariableName=u_device_Q1_ideal_inv_sim  SampleTime=tc
      settings: MaxDataPoints=Nc
  To Workspace4 : ToWorkspace  VariableName=us_inv_modA_sim  SampleTime=tc
      settings: MaxDataPoints=Nc
  To Workspace40 : ToWorkspace  VariableName=i_device_Q2_ideal_zvs_sim  SampleTime=tc
      settings: MaxDataPoints=Nc
  To Workspace41 : ToWorkspace  VariableName=i_device_Q2_ideal_inv_sim  SampleTime=tc
      settings: MaxDataPoints=Nc
  To Workspace42 : ToWorkspace  VariableName=u_device_Q2_ideal_zvs_sim  SampleTime=tc
      settings: MaxDataPoints=Nc
  To Workspace43 : ToWorkspace  VariableName=u_device_Q2_ideal_inv_sim  SampleTime=tc
      settings: MaxDataPoints=Nc
  To Workspace44 : ToWorkspace  VariableName=u_device_Q1_mosfet_zvs_sim  SampleTime=tc
      settings: MaxDataPoints=Nc
  To Workspace45 : ToWorkspace  VariableName=u_device_Q1_mosfet_inv_sim  SampleTime=tc
      settings: MaxDataPoints=Nc
  To Workspace46 : ToWorkspace  VariableName=i_device_Q2_mosfet_zvs_sim  SampleTime=tc
      settings: MaxDataPoints=Nc
  To Workspace47 : ToWorkspace  VariableName=i_device_Q2_mosfet_inv_sim  SampleTime=tc
      settings: MaxDataPoints=Nc
  To Workspace48 : ToWorkspace  VariableName=u_device_Q2_mosfet_zvs_sim  SampleTime=tc
      settings: MaxDataPoints=Nc
  To Workspace49 : ToWorkspace  VariableName=u_device_Q2_mosfet_inv_sim  SampleTime=tc
      settings: MaxDataPoints=Nc
  To Workspace5 : ToWorkspace  VariableName=dc_bus_terminal_current_inverter_sim  SampleTime=tc
      settings: MaxDataPoints=Nc
  To Workspace50 : ToWorkspace  VariableName=dclink_voltage_inverter_modA_sim  SampleTime=tc
      settings: MaxDataPoints=Nc
  To Workspace51 : ToWorkspace  VariableName=CFu_dc_voltage_sim  SampleTime=tc
      settings: MaxDataPoints=Nc
  To Workspace52 : ToWorkspace  VariableName=zvs_current_output_modA_sim  SampleTime=tc
      settings: MaxDataPoints=Nc
  To Workspace53 : ToWorkspace  VariableName=zvs_voltage_output_modA_sim  SampleTime=tc
      settings: MaxDataPoints=Nc
  To Workspace54 : ToWorkspace  VariableName=u_diode_rectifier_sim  SampleTime=tc
      settings: MaxDataPoints=Nc
  To Workspace6 : ToWorkspace  VariableName=CFi_dc_current_sim  SampleTime=tc
      settings: MaxDataPoints=Nc
  To Workspace7 : ToWorkspace  VariableName=CFi_dc_voltage_sim  SampleTime=tc
      settings: MaxDataPoints=Nc
  To Workspace8 : ToWorkspace  VariableName=Cs_voltage_sim  SampleTime=tc
      settings: MaxDataPoints=Nc
  To Workspace9 : ToWorkspace  VariableName=Ls_current_sim  SampleTime=tc
      settings: MaxDataPoints=Nc
  wires:
  Clock/1 -> To Workspace1/1
  [inverter_current_output_modA] -> To Workspace16/1
  [inverter_voltage_output_modA] -> To Workspace2/1
  [is_inv_modA] -> To Workspace3/1
  [us_inv_modA] -> To Workspace4/1
  [dc_bus_terminal_current_inverter] -> To Workspace5/1
  [CFi_dc_current] -> To Workspace6/1
  [dab_voltage_input_modA] -> To Workspace7/1
  [Cs_voltage] -> To Workspace8/1
  [Ls_current] -> To Workspace9/1
  [CFu_ac_current] -> To Workspace10/1
  [is_inv_modA] -> To Workspace11/1
  [u1_hf_trafo] -> To Workspace12/1
  [LFu1_dc_current] -> To Workspace13/1
  [voltage_battery] -> To Workspace14/1
  [current_battery] -> To Workspace15/1
  [mosfet_JH_temp_zvs] -> To Workspace17/1
  [mosfet_HA_temp_zvs] -> To Workspace18/1
  [mosfet_power_losses_zvs] -> To Workspace19/1
  [mosfet_power_losses_inv] -> To Workspace22/1
  [mosfet_HA_temp_inv] -> To Workspace21/1
  [mosfet_JH_temp_inv] -> To Workspace20/1
  [CFi_dc2_current_modA] -> To Workspace23/1
  [i_device_Q1_ideal_zvs] -> To Workspace24/1
  [i_device_Q1_thermal_zvs] -> To Workspace25/1
  [i_device_Q1_mosfet_zvs] -> To Workspace26/1
  [i_device_Q1_mosfet_inv] -> To Workspace29/1
  [i_device_Q1_ideal_inv] -> To Workspace27/1
  [u_tr2_out] -> To Workspace30/1
  [i_tr2_out] -> To Workspace31/1
  [u_device_Q1_thermal_zvs] -> To Workspace32/1
  [u_device_Q2_thermal_zvs] -> To Workspace34/1
  [i_device_Q2_thermal_zvs] -> To Workspace33/1
  [i_device_Q2_thermal_inv] -> To Workspace37/1
  [u_device_Q2_thermal_inv] -> To Workspace38/1
  [u_device_Q1_thermal_inv] -> To Workspace36/1
  [i_device_Q1_thermal_inv] -> To Workspace35/1
  [u_device_Q1_ideal_zvs] -> To Workspace28/1
  [u_device_Q1_ideal_inv] -> To Workspace39/1
  [u_device_Q2_ideal_inv] -> To Workspace43/1
  [u_device_Q2_ideal_zvs] -> To Workspace42/1
  [i_device_Q2_ideal_inv] -> To Workspace41/1
  [i_device_Q2_ideal_zvs] -> To Workspace40/1
  [u_device_Q1_mosfet_inv] -> To Workspace45/1
  [u_device_Q1_mosfet_zvs] -> To Workspace44/1
  [u_device_Q2_mosfet_zvs] -> To Workspace48/1
  [u_device_Q2_mosfet_inv] -> To Workspace49/1
  [i_device_Q2_mosfet_inv] -> To Workspace47/1
  [i_device_Q2_mosfet_zvs] -> To Workspace46/1
  [dclink_voltage_inverter_modA] -> To Workspace50/1
  [CFi_dc2_voltage] -> To Workspace51/1
  [dab_voltage_output_modA] -> To Workspace53/1
  [dab_current_output_modA] -> To Workspace52/1
  [u_diode_rectifier] -> To Workspace54/1

== system sst/battery/LithiumIonBattery ==
  Current Sensor : fl_lib/Electrical/Electrical Sensors/Current Sensor
  Electrical Reference1 : fl_lib/Electrical/Electrical Elements/Electrical Reference
  PS-Simulink Converter4 : nesl_utility/PS-Simulink Converter  PhysicalDomain=network_engine_domain  SubClassName=ps_output  LeftPortType=input  RightPortType=output  PseudoPeriodic=off  Frequencies=[]  VectorFormat=1-D array  Unit=1  AffineConversion=off
  PS-Simulink Converter5 : nesl_utility/PS-Simulink Converter  PhysicalDomain=network_engine_domain  SubClassName=ps_output  LeftPortType=input  RightPortType=output  PseudoPeriodic=off  Frequencies=[]  VectorFormat=1-D array  Unit=V  AffineConversion=on
  SOC_estimator : Subsystem
  To Workspace1 : ToWorkspace  VariableName=idc_battery_sim  SampleTime=tc
      settings: MaxDataPoints=Nc
  To Workspace2 : ToWorkspace  VariableName=udc_battery_sim  SampleTime=tc
      settings: MaxDataPoints=Nc
  Unit Delay5 : UnitDelay  SampleTime=ts_battery  HasFrameUpgradeWarning=on
  Voltage Sensor : fl_lib/Electrical/Electrical Sensors/Voltage Sensor
  ibat/vdc : Scope  NumInputPorts=2
      settings: SampleTime=tc  ActiveDisplayYMinimum=-188.41234320293574  ActiveDisplayYMaximum=402.735491049541  DataLoggingVariableName=ScopeData6
  lithium ion cell analytical ocv : Subsystem
  Uout+ : PMIOPort  Side=Right
  Uout- : PMIOPort  Port=2  Side=Right
  wires:
  PS-Simulink Converter5/1 -> Unit Delay5/1
  PS-Simulink Converter4/1 -> To Workspace1/1, ibat/vdc/1  "i batt"
  Unit Delay5/1 -> To Workspace2/1, [vdc]
  [vdc] -> ibat/vdc/2  "vdc"
  connections:
  Current Sensor/RConn1 -- PS-Simulink Converter4/LConn1
  Uout+/RConn1 -- Current Sensor/RConn2 -- Voltage Sensor/LConn1
  Voltage Sensor/RConn1 -- PS-Simulink Converter5/LConn1
  Voltage Sensor/RConn2 -- Electrical Reference1/LConn1 -- lithium ion cell analytical ocv/RConn2 -- Uout-/RConn1
  lithium ion cell analytical ocv/RConn1 -- Current Sensor/LConn1

== system sst/dab_modA/dab_ctrl ==
  Bus Creator : BusCreator  Inputs=8
  modulator1 : Subsystem
  references : Subsystem
  sampling_i_filter1 : Subsystem
  sampling_v_filter1 : Subsystem
  sampling_v_filter2 : Subsystem
  vi ctrl : Subsystem
  gate_commands : Outport
  wires:
  [dab_voltage_output_modA] -> sampling_v_filter1/1(in)
  [i_dab_input_modA] -> sampling_i_filter1/1(in)
  vi ctrl/1(phase_displacement) -> modulator1/1(phase_displacement)
  sampling_i_filter1/1(out_pu) -> vi ctrl/1(i_dab_input)
  sampling_v_filter1/1(out_pu) -> vi ctrl/2(u_dab_output)
  sampling_v_filter2/1(out_pu) -> vi ctrl/3(u_dab_output_ref)
  references/1(vout_ref) -> sampling_v_filter2/1(in)
  Bus Creator/1 -> gate_commands/1
  modulator1/1(gate_Q1) -> Bus Creator/1
  modulator1/2(gate_Q2) -> Bus Creator/2
  modulator1/3(gate_Q3) -> Bus Creator/3
  modulator1/4(gate_Q4) -> Bus Creator/4
  modulator1/5(gate_Q5) -> Bus Creator/5
  modulator1/6(gate_Q6) -> Bus Creator/6
  modulator1/7(gate_Q7) -> Bus Creator/7
  modulator1/8(gate_Q8) -> Bus Creator/8

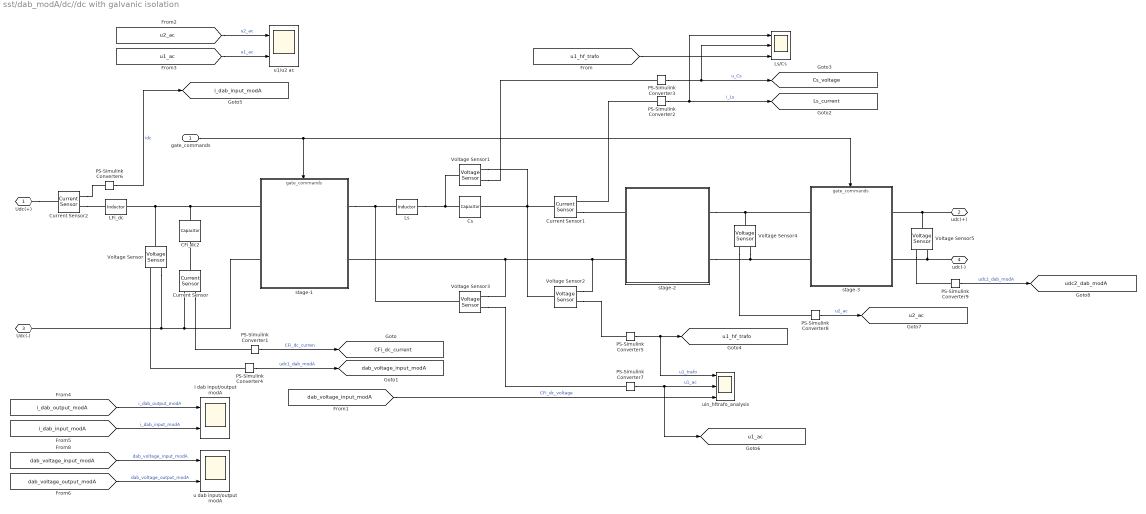
== system sst/dab_modA/dc//dc with galvanic isolation ==
  gate_commands : Inport
  CFi_dc2 : fl_lib/Electrical/Electrical Elements/Capacitor  c=CFi_dc1 F  r=RCFi_dc1_internal Ohm  g=0 1/Ohm  i_specify=off  i_priority=None  i=0 A  i_nominal_specify=off  i_nominal_value=1  i_nominal_unit=A  v_specify=off  v_priority=None  v=0 V  v_nominal_specify=off  v_nominal_value=1  v_nominal_unit=V  vc_specify=off  vc_priority=High  vc=0 V  vc_nominal_specify=off  vc_nominal_value=1  vc_nominal_unit=V
  Cs : fl_lib/Electrical/Electrical Elements/Capacitor  c=Cs1 F  r=1e-6 Ohm  g=0 1/Ohm  i_specify=off  i_priority=None  i=0 A  i_nominal_specify=off  i_nominal_value=1  i_nominal_unit=A  v_specify=off  v_priority=None  v=0 V  v_nominal_specify=off  v_nominal_value=1  v_nominal_unit=V  vc_specify=off  vc_priority=High  vc=0 V  vc_nominal_specify=off  vc_nominal_value=1  vc_nominal_unit=V
  Current Sensor : fl_lib/Electrical/Electrical Sensors/Current Sensor
  Current Sensor1 : fl_lib/Electrical/Electrical Sensors/Current Sensor
  Current Sensor2 : fl_lib/Electrical/Electrical Sensors/Current Sensor
  LFi_dc : fl_lib/Electrical/Electrical Elements/Inductor  l=LFi_dc H  r=RLFi_dc Ohm  g=1e-9 1/Ohm  i_specify=off  i_priority=None  i=0 A  i_nominal_specify=off  i_nominal_value=1  i_nominal_unit=A  v_specify=off  v_priority=None  v=0 V  v_nominal_specify=off  v_nominal_value=1  v_nominal_unit=V  i_L_specify=off  i_L_priority=High  i_L=0 A  i_L_nominal_specify=off  i_L_nominal_value=1  i_L_nominal_unit=A
  Ls : fl_lib/Electrical/Electrical Elements/Inductor  l=Ls1 H  r=0 Ohm  g=1e-9 1/Ohm  i_specify=off  i_priority=None  i=0 A  i_nominal_specify=off  i_nominal_value=1  i_nominal_unit=A  v_specify=off  v_priority=None  v=0 V  v_nominal_specify=off  v_nominal_value=1  v_nominal_unit=V  i_L_specify=off  i_L_priority=High  i_L=0 A  i_L_nominal_specify=off  i_L_nominal_value=1  i_L_nominal_unit=A
  Ls/Cs : Scope  NumInputPorts=3
      settings: SampleTime=tc  ActiveDisplayYMinimum=-8555.37696713307  ActiveDisplayYMaximum=8509.29404508231
  PS-Simulink Converter1 : nesl_utility/PS-Simulink Converter  PhysicalDomain=network_engine_domain  SubClassName=ps_output  LeftPortType=input  RightPortType=output  PseudoPeriodic=off  Frequencies=[]  VectorFormat=1-D array  Unit=A  AffineConversion=on
  PS-Simulink Converter2 : nesl_utility/PS-Simulink Converter  PhysicalDomain=network_engine_domain  SubClassName=ps_output  LeftPortType=input  RightPortType=output  PseudoPeriodic=off  Frequencies=[]  VectorFormat=1-D array  Unit=A  AffineConversion=on
  PS-Simulink Converter{3..5,7..9} (6 alike) : nesl_utility/PS-Simulink Converter  PhysicalDomain=network_engine_domain  SubClassName=ps_output  LeftPortType=input  RightPortType=output  PseudoPeriodic=off  Frequencies=[]  VectorFormat=1-D array  Unit=V  AffineConversion=on
  PS-Simulink Converter6 : nesl_utility/PS-Simulink Converter  PhysicalDomain=network_engine_domain  SubClassName=ps_output  LeftPortType=input  RightPortType=output  PseudoPeriodic=off  Frequencies=[]  VectorFormat=1-D array  Unit=A  AffineConversion=on
  Voltage Sensor{,1..5} (6 alike) : fl_lib/Electrical/Electrical Sensors/Voltage Sensor
  i dab input/output modA : Scope  NumInputPorts=2
      settings: SampleTime=tc  ActiveDisplayYMinimum=-3745.5802333321844  ActiveDisplayYMaximum=2860.9744612967625  DataLoggingVariableName=ScopeData8
  stage-1 : Subsystem
      settings: PortSchema="{\"entries\":[{\"content\":{\"sides\":[{\"content\":{\"connectorIds\":[\"LConn1\",\"LConn2\"]},\"type\":\"ConnectorPlacement.EquallySpacedRectSide\",\"uuid\":\"c872503a-61af-4937-bdf2-4de4f8645573\"},{\"content\":{\"connectorIds\":[\"RConn1\",\"RConn2\"],\"side\":\"RIGHT\"},\"type\":\"ConnectorPlacement.EquallySpacedRectSide\",\"uuid\":\"3b83f060-86a2-4569-84b5-d9f7c0485347\"},{\"content\":{\"connectorIds\":[\"In1\"],\"side\":\"TOP\"},\"type\":\"ConnectorPlacement.EquallySpacedRectSide\",\"uuid\":\"bf191d46-ce71-4d15-9dd0-24cc57253577\"}]},\"type\":\"ConnectorPlacement.EquallySpacedConnector\",\"uuid\":\"1b28ceee-25d0-45ae-a3c4-c2563f0d63ba\"}],\"packageUris\":[\"http://schema.mathworks.com/mf0/Connector/R2020b\"],\"version\":\"1.0\"}"
  stage-2 : Subsystem
  stage-3 : Subsystem
      settings: PortSchema="{\"entries\":[{\"content\":{\"sides\":[{\"content\":{\"connectorIds\":[\"LConn1\",\"LConn2\"]},\"type\":\"ConnectorPlacement.EquallySpacedRectSide\",\"uuid\":\"c872503a-61af-4937-bdf2-4de4f8645573\"},{\"content\":{\"connectorIds\":[\"RConn1\",\"RConn2\"],\"side\":\"RIGHT\"},\"type\":\"ConnectorPlacement.EquallySpacedRectSide\",\"uuid\":\"3b83f060-86a2-4569-84b5-d9f7c0485347\"},{\"content\":{\"connectorIds\":[\"In1\"],\"side\":\"TOP\"},\"type\":\"ConnectorPlacement.EquallySpacedRectSide\",\"uuid\":\"bf191d46-ce71-4d15-9dd0-24cc57253577\"}]},\"type\":\"ConnectorPlacement.EquallySpacedConnector\",\"uuid\":\"1b28ceee-25d0-45ae-a3c4-c2563f0d63ba\"}],\"packageUris\":[\"http://schema.mathworks.com/mf0/Connector/R2020b\"],\"version\":\"1.0\"}"
  u dab input/output modA : Scope  NumInputPorts=2
      settings: SampleTime=tc  ActiveDisplayYMinimum=-2317.3160340943446  ActiveDisplayYMaximum=22315.278521944136  DataLoggingVariableName=ScopeData10
  u1/u2 ac : Scope  NumInputPorts=2
      settings: SampleTime=tc  ActiveDisplayYMinimum=-24809.384739578214  ActiveDisplayYMaximum=24819.433595470524  DataLoggingVariableName=ScopeData5
  uin_hftrafo_analysis : Scope  NumInputPorts=3
      settings: SampleTime=tc  ActiveDisplayYMinimum=-13659.242458711054  ActiveDisplayYMaximum=12378.723081515578
  Udc(+) : PMIOPort  Side=Left
  udc(+) : PMIOPort  Port=2  Side=Right
  Udc(-) : PMIOPort  Port=3  Side=Left
  udc(-) : PMIOPort  Port=4  Side=Right
  tag scope: CFi_dc_current=global, Cs_voltage=global, Ls_current=global, dab_voltage_input_modA=global, i_dab_input_modA=global, u1_ac=global, u1_hf_trafo=global, u2_ac=global, udc2_dab_modA=global
  wires:
  gate_commands/1 -> stage-3/1(gate_commands), stage-1/1(gate_commands)
  PS-Simulink Converter1/1 -> [CFi_dc_current]  "CFi_dc_curren"
  PS-Simulink Converter4/1 -> [dab_voltage_input_modA]  "udc1_dab_modA"
  PS-Simulink Converter2/1 -> Ls/Cs/1, [Ls_current]  "i_Ls"
  PS-Simulink Converter3/1 -> Ls/Cs/2, [Cs_voltage]  "u_Cs"
  PS-Simulink Converter5/1 -> uin_hftrafo_analysis/1, [u1_hf_trafo]  "u1_trafo"
  [u1_hf_trafo] -> Ls/Cs/3
  PS-Simulink Converter7/1 -> [u1_ac], uin_hftrafo_analysis/2  "u1_ac"
  [dab_voltage_input_modA] -> uin_hftrafo_analysis/3  "CFi_dc_voltage"
  PS-Simulink Converter6/1 -> [i_dab_input_modA]  "idc"
  PS-Simulink Converter8/1 -> [u2_ac]  "u2_ac"
  [u2_ac] -> u1/u2 ac/1  "u2_ac"
  [u1_ac] -> u1/u2 ac/2  "u1_ac"
  [i_dab_input_modA] -> i dab input/output modA/2  "i_dab_input_modA"
  [i_dab_output_modA] -> i dab input/output modA/1  "i_dab_output_modA"
  PS-Simulink Converter9/1 -> [udc2_dab_modA]  "udc2_dab_modA"
  [dab_voltage_input_modA] -> u dab input/output modA/1  "dab_voltage_input_modA"
  [dab_voltage_output_modA] -> u dab input/output modA/2  "dab_voltage_output_modA"
  connections:
  stage-2/LConn2 -- Voltage Sensor2/RConn2 -- stage-1/LConn2 -- Voltage Sensor3/RConn2
  stage-1/RConn1 -- CFi_dc2/LConn1 -- LFi_dc/RConn1 -- Voltage Sensor/LConn1
  stage-1/RConn2 -- Current Sensor/RConn2 -- Udc(-)/RConn1 -- Voltage Sensor/RConn2
  Current Sensor/LConn1 -- CFi_dc2/RConn1
  Current Sensor/RConn1 -- PS-Simulink Converter1/LConn1
  PS-Simulink Converter4/LConn1 -- Voltage Sensor/RConn1
  stage-1/LConn1 -- Voltage Sensor3/LConn1 -- Ls/LConn1
  Current Sensor1/RConn2 -- stage-2/LConn1
  PS-Simulink Converter2/LConn1 -- Current Sensor1/RConn1
  Voltage Sensor1/RConn1 -- PS-Simulink Converter3/LConn1
  Voltage Sensor2/RConn1 -- PS-Simulink Converter5/LConn1
  Voltage Sensor1/RConn2 -- Current Sensor1/LConn1 -- Cs/RConn1 -- Voltage Sensor2/LConn1
  Ls/RConn1 -- Cs/LConn1 -- Voltage Sensor1/LConn1
  Voltage Sensor3/RConn1 -- PS-Simulink Converter7/LConn1
  stage-2/RConn1 -- Voltage Sensor4/LConn1 -- stage-3/LConn1
  stage-2/RConn2 -- Voltage Sensor4/RConn2 -- stage-3/LConn2
  udc(+)/RConn1 -- Voltage Sensor5/LConn1 -- stage-3/RConn1
  udc(-)/RConn1 -- Voltage Sensor5/RConn2 -- stage-3/RConn2
  Current Sensor2/RConn2 -- LFi_dc/LConn1
  Udc(+)/RConn1 -- Current Sensor2/LConn1
  Current Sensor2/RConn1 -- PS-Simulink Converter6/LConn1
  Voltage Sensor4/RConn1 -- PS-Simulink Converter8/LConn1
  Voltage Sensor5/RConn1 -- PS-Simulink Converter9/LConn1

== system sst/dab_modA/single_phase_ui_measure1 ==
  Bus Creator : BusCreator  Inputs=2
  Current Sensor : fl_lib/Electrical/Electrical Sensors/Current Sensor
  Selector : Selector  InputPortWidth=2  IndexOptions=Index vector (dialog)  Indices=2  OutputSizes=1
  Selector1 : Selector  InputPortWidth=2  IndexOptions=Index vector (dialog)  Indices=1  OutputSizes=1
  Voltage Sensor : fl_lib/Electrical/Electrical Sensors/Voltage Sensor
  dab input modA : Scope  NumInputPorts=2
      settings: SampleTime=tc  ActiveDisplayYMinimum=-479.16980062874819  ActiveDisplayYMaximum=409.04253534221243  DataLoggingVariableName=ScopeData2
  iph : nesl_utility/PS-Simulink Converter  PhysicalDomain=network_engine_domain  SubClassName=ps_output  LeftPortType=input  RightPortType=output  PseudoPeriodic=off  Frequencies=[]  VectorFormat=1-D array  Unit=A  AffineConversion=off
  uph : nesl_utility/PS-Simulink Converter  PhysicalDomain=network_engine_domain  SubClassName=ps_output  LeftPortType=input  RightPortType=output  PseudoPeriodic=off  Frequencies=[]  VectorFormat=1-D array  Unit=V  AffineConversion=off
  Udc(+) : PMIOPort  Side=Left
  udc(+) : PMIOPort  Port=2  Side=Right
  Udc(-) : PMIOPort  Port=3  Side=Left
  udc(-) : PMIOPort  Port=4  Side=Right
  tag scope: current_battery=global, voltage_battery=global
  wires:
  Bus Creator/1 -> Selector/1, Selector1/1  "ui_data"
  iph/1 -> Bus Creator/1  "iph"
  uph/1 -> Bus Creator/2  "uph"
  Selector1/1 -> [current_battery], dab input modA/1  "current_battery"
  Selector/1 -> dab input modA/2, [voltage_battery]  "voltage_battery"
  connections:
  iph/LConn1 -- Current Sensor/RConn1
  Voltage Sensor/LConn1 -- Current Sensor/LConn1 -- Udc(+)/RConn1
  Current Sensor/RConn2 -- udc(+)/RConn1
  Voltage Sensor/RConn1 -- uph/LConn1
  Voltage Sensor/RConn2 -- Udc(-)/RConn1 -- udc(-)/RConn1

== system sst/dab_modA/ui_measure ==
  Bus Creator : BusCreator  Inputs=2
  Current Sensor : fl_lib/Electrical/Electrical Sensors/Current Sensor
  Selector : Selector  InputPortWidth=2  IndexOptions=Index vector (dialog)  Indices=2  OutputSizes=1
  Selector1 : Selector  InputPortWidth=2  IndexOptions=Index vector (dialog)  Indices=1  OutputSizes=1
  Voltage Sensor : fl_lib/Electrical/Electrical Sensors/Voltage Sensor
  dab output modA : Scope  NumInputPorts=2
      settings: SampleTime=tc  ActiveDisplayYMinimum=-347219.58035464212  ActiveDisplayYMaximum=2.5921819118290781E+6  DataLoggingVariableName=ScopeData2
  iph : nesl_utility/PS-Simulink Converter  PhysicalDomain=network_engine_domain  SubClassName=ps_output  LeftPortType=input  RightPortType=output  PseudoPeriodic=off  Frequencies=[]  VectorFormat=1-D array  Unit=A  AffineConversion=off
  uph : nesl_utility/PS-Simulink Converter  PhysicalDomain=network_engine_domain  SubClassName=ps_output  LeftPortType=input  RightPortType=output  PseudoPeriodic=off  Frequencies=[]  VectorFormat=1-D array  Unit=V  AffineConversion=off
  Udc(+) : PMIOPort  Side=Left
  udc(+) : PMIOPort  Port=2  Side=Right
  Udc(-) : PMIOPort  Port=3  Side=Left
  udc(-) : PMIOPort  Port=4  Side=Right
  tag scope: dab_current_output_modA=global, dab_voltage_output_modA=global
  wires:
  [dab_current_output_modA] -> dab output modA/1  "dab_current_output_modA"
  [dab_voltage_output_modA] -> dab output modA/2  "dab_voltage_output_modA"
  Selector1/1 -> [dab_current_output_modA]
  Selector/1 -> [dab_voltage_output_modA]
  Bus Creator/1 -> Selector/1, Selector1/1  "ui_data"
  iph/1 -> Bus Creator/1  "iph"
  uph/1 -> Bus Creator/2  "uph"
  connections:
  iph/LConn1 -- Current Sensor/RConn1
  Voltage Sensor/LConn1 -- Current Sensor/LConn1 -- Udc(+)/RConn1
  Current Sensor/RConn2 -- udc(+)/RConn1
  Voltage Sensor/RConn1 -- uph/LConn1
  Voltage Sensor/RConn2 -- Udc(-)/RConn1 -- udc(-)/RConn1

== system sst/dab_modB/dab_ctrl ==
  Bus Creator : BusCreator  Inputs=8
  modulator1 : Subsystem
  references : Subsystem
  sampling_i_filter1 : Subsystem
  sampling_v_filter1 : Subsystem
  sampling_v_filter2 : Subsystem
  vi ctrl : Subsystem
  gate_commands : Outport
  wires:
  modulator1/8(gate_Q8) -> Bus Creator/8
  modulator1/7(gate_Q7) -> Bus Creator/7
  modulator1/6(gate_Q6) -> Bus Creator/6
  modulator1/5(gate_Q5) -> Bus Creator/5
  modulator1/4(gate_Q4) -> Bus Creator/4
  modulator1/3(gate_Q3) -> Bus Creator/3
  modulator1/2(gate_Q2) -> Bus Creator/2
  modulator1/1(gate_Q1) -> Bus Creator/1
  Bus Creator/1 -> gate_commands/1
  references/1(vout_ref) -> sampling_v_filter2/1(in)
  sampling_v_filter2/1(out_pu) -> vi ctrl/3(u_dab_output_ref)
  sampling_v_filter1/1(out_pu) -> vi ctrl/2(u_dab_output)
  sampling_i_filter1/1(out_pu) -> vi ctrl/1(i_dab_input)
  vi ctrl/1(phase_displacement) -> modulator1/1(phase_displacement)
  [i_dab_input_modB] -> sampling_i_filter1/1(in)
  [dab_voltage_output_modB] -> sampling_v_filter1/1(in)
